simulink model "third"  (R2023b)
settings: Solver=FixedStepAuto  StartTime=0.0  StopTime=10  FixedStep=0.0001  RelTol=1e-3
libraries: dspsrcs4 x2
settings Model: Creator=evdokiiagalkina  LastModifiedBy=evdokiiagalkina

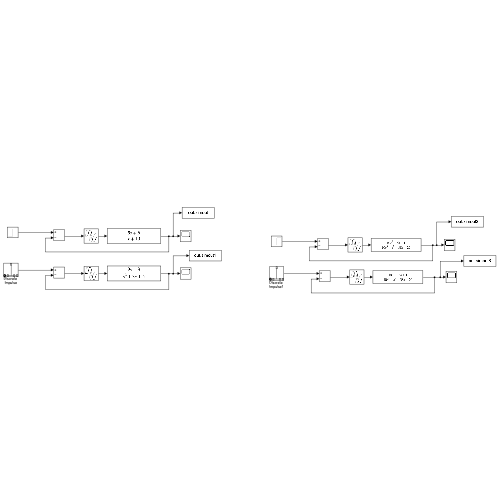
[thumbnail: Simulink's stored preview of the top-level diagram]
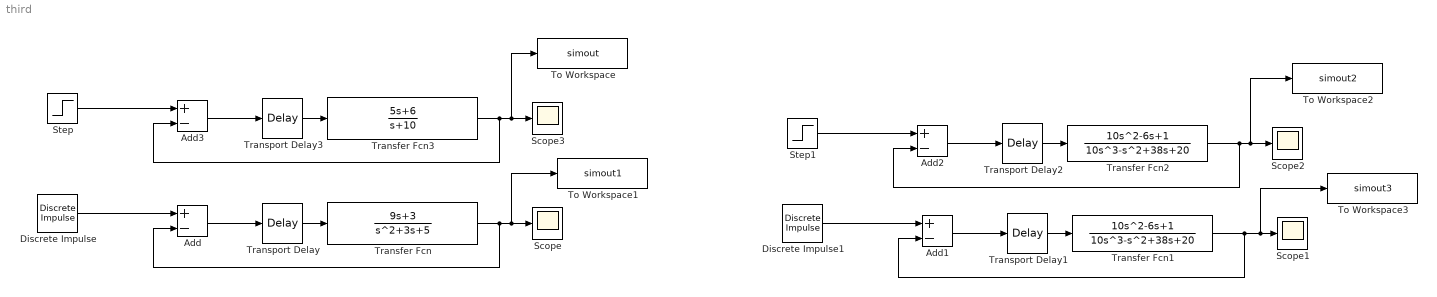
== system third ==
  Add{,1..3} (4 alike) : Sum  Inputs=+-
  Discrete Impulse : dspsrcs4/Discrete  Impulse  Delay=0  SampleTime=1  FrameSample=1  OutputFrames=off  dataType=double  isSigned=on  wordLen=16  udDataType=sfix(16)  fracBitsMode=Best precision  numFracBits=15  OutDataTypeStr=double  LastOutDataTypeStr=double
  Discrete Impulse1 : dspsrcs4/Discrete  Impulse  Delay=0  SampleTime=1  FrameSample=1  OutputFrames=off  dataType=double  isSigned=on  wordLen=16  udDataType=sfix(16)  fracBitsMode=Best precision  numFracBits=15  OutDataTypeStr=double  LastOutDataTypeStr=double
  Scope{,1..3} (4 alike) : Scope
  Step : Step  SampleTime=0
  Step1 : Step  SampleTime=0
  To Workspace : ToWorkspace  VariableName=simout  SaveFormat=Timeseries  SampleTime=-1
  To Workspace1 : ToWorkspace  VariableName=simout1  SaveFormat=Timeseries  SampleTime=-1
  To Workspace2 : ToWorkspace  VariableName=simout2  SaveFormat=Timeseries  SampleTime=-1
  To Workspace3 : ToWorkspace  VariableName=simout3  SaveFormat=Timeseries  SampleTime=-1
  Transfer Fcn : TransferFcn  Numerator=[9 3]  Denominator=[1 3 5]
  Transfer Fcn1 : TransferFcn  Numerator=[10 -6 1]  Denominator=[10 -1 38 20]
  Transfer Fcn2 : TransferFcn  Numerator=[10 -6 1]  Denominator=[10 -1 38 20]
  Transfer Fcn3 : TransferFcn  Numerator=[5 6]  Denominator=[1 10]
  Transport Delay : TransportDelay
  Transport Delay1 : TransportDelay  DelayTime=5
  Transport Delay2 : TransportDelay  DelayTime=5
  Transport Delay3 : TransportDelay  DelayTime=0.1
  wires:
  Transfer Fcn/1 -> To Workspace1/1, Scope/1, Add/2
  Transport Delay/1 -> Transfer Fcn/1
  Add/1 -> Transport Delay/1
  Discrete Impulse/1 -> Add/1
  Transfer Fcn1/1 -> Add1/2, To Workspace3/1, Scope1/1
  Transport Delay1/1 -> Transfer Fcn1/1
  Add1/1 -> Transport Delay1/1
  Discrete Impulse1/1 -> Add1/1
  Add2/1 -> Transport Delay2/1
  Step1/1 -> Add2/1
  Transport Delay2/1 -> Transfer Fcn2/1
  Transfer Fcn2/1 -> Add2/2, To Workspace2/1, Scope2/1
  Transfer Fcn3/1 -> To Workspace/1, Scope3/1, Add3/2
  Transport Delay3/1 -> Transfer Fcn3/1
  Add3/1 -> Transport Delay3/1
  Step/1 -> Add3/1
